simulink model "roach2_fengine_nlb"  (R2013b)
settings: Solver=VariableStepDiscrete  SolverMode=SingleTasking  StartTime=0.0  StopTime=10.0  RelTol=1e-3
undefined symbols (not defined in the file or in its folder): sfp
libraries: xbsIndex_r4 x3316, xps_library x74, casper_library_sources x16, casper_library_misc x7
(part 1 of 38)
settings Model: Creator=mdexter  LastModifiedBy=jackh
settings DataIOCC: SignalLoggingSaveFormat=ModelDataLogs
settings OptimizationCC: InlineParams=on  ExpressionDepthLimit=2147483647
settings DebuggingCC: FcnCallInpInsideContextMsg=UseLocalSettings  StateNameClashWarn=warning
settings GRTTargetCC: CombineOutputUpdateFcns=off  GRTInterface=on

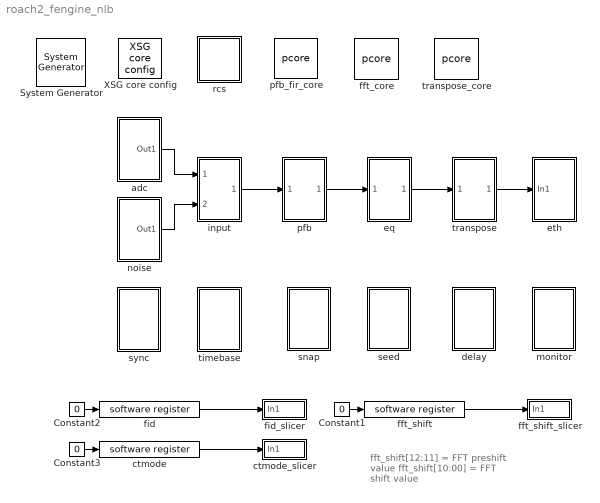
== system roach2_fengine_nlb ==
  note: fft_shift[12:11] = FFT preshift value
      | fft_shift[10:00] = FFT shift value
  " System Generator" : xbsIndex_r4/ System Generator  Tag=genX  xilinxfamily=virtex6  part=xc6vsx475t  speed=-1  package=ff1759  synthesis_tool=XST  clock_wrapper=Clock Enables  directory=./roach2_fengine/sysgen  proj_type=Project Navigator  Synth_file=XST Defaults  Impl_file=ISE Defaults  testbench=off  simulink_period=1  sysclk_period=5  dcm_input_clock_period=100  incr_netlist=off  trim_vbits=Everywhere in SubSystem  dbl_ovrd=According to Block Masks  core_generation=According to Block Masks  run_coregen=off  deprecated_control=off  eval_field=0  block_type=sysgen
      settings: block_version=10.1.3
  Constant1 : Constant  Value=0
  Constant2 : Constant  Value=0
  Constant3 : Constant  Value=0
  XSG core config : xps_library/XSG core config  Tag=xps:xsg  hw_sys=ROACH2:sx475t  clk_src=adc0_clk  ROACH_clk_src=adc0_clk  ROACH2_clk_src=adc0_clk  clk_rate=200  sample_period=1  synthesis_tool=XST
  adc : Subsystem
  ctmode : xps_library/software register  Tag=xps:sw_reg  io_dir=From Processor  arith_type=Unsigned  bitwidth=32  bin_pt=0  sample_period=1  gw_name=roach2_fengine_orig_ctmode_user_data_out
  ctmode_slicer : Subsystem
  delay : Subsystem
  eq : Subsystem
  eth : Subsystem
  fft_core : xps_library/pcore  Tag=xps:pcore  pcore_path=fft_1024ch_core/fft_1024ch_core.ngc
  fft_shift : xps_library/software register  Tag=xps:sw_reg  io_dir=From Processor  arith_type=Unsigned  bitwidth=32  bin_pt=0  sample_period=1  gw_name=roach2_fengine_orig_fft_shift_user_data_out
  fft_shift_slicer : Subsystem
  fid : xps_library/software register  Tag=xps:sw_reg  io_dir=From Processor  arith_type=Unsigned  bitwidth=32  bin_pt=0  sample_period=1  gw_name=roach2_fengine_orig_fid_user_data_out
  fid_slicer : Subsystem
  input : Subsystem
  monitor : Subsystem
  noise : Subsystem
  pfb : Subsystem
  pfb_fir_core : xps_library/pcore  Tag=xps:pcore  pcore_path=pfb_fir_1024ch_core/pfb_fir_1024ch_core.ngc
  rcs : Subsystem  AncestorBlock=casper_library_misc/rcs  mask(rcs){app_src=git, lib_src=git, user_val=0}
      mask prompts: app_src "Application revision info to capture"; lib_src "CASPER libraries revision info to capture"; user_val "User specified value"
      mask help:
      | Embeds revision control information for the user design and libraries.
      | On failure to locate specified revision information, falls back to
      | timestamps (current time for libraries).
      | A user specified value is also stored.
      mask init:
      | rcs_init(gcb, ...
      |     'app_src', app_src, ...
      |     'lib_src', lib_src);
      mask TypeOptions app_src: timestamp | git | svn
      mask TypeOptions lib_src: timestamp | git | svn
  seed : Subsystem
  snap : Subsystem
  sync : Subsystem
  timebase : Subsystem
  transpose : Subsystem
  transpose_core : xps_library/pcore  Tag=xps:pcore  pcore_path=transpose_core/transpose_core.ngc
  wires:
  input/1(Out1) -> pfb/1(In1)
  pfb/1(Out1) -> eq/1(In1)
  eq/1(Out2) -> transpose/1(In1)
  adc/1(Out1) -> input/1(In1)
  noise/1(Out1) -> input/2(In2)
  transpose/1(Out1) -> eth/1(In1)
  fft_shift/1 -> fft_shift_slicer/1(In1)
  Constant1/1 -> fft_shift/1
  fid/1 -> fid_slicer/1(In1)
  Constant2/1 -> fid/1
  ctmode/1 -> ctmode_slicer/1(In1)
  Constant3/1 -> ctmode/1

== system roach2_fengine_nlb/adc ==
  Bus Creator : BusCreator  Inputs=32
  Constant{3..34} (32 alike) : Constant  Value=0
  adc16x250-8 : Subsystem  Tag=xps:adc16  AncestorBlock=xps_library/ADCs/adc16x250-8  mask(ADC16){board_count=2, roach2_rev=2, zdok_rev=2}
      mask prompts: board_count "Number of ADC16 Boards"; roach2_rev "ROACH2 Revision"; zdok_rev "ZDOK Pinout Revision"
      mask help: 16-input ADC. When using one ADC16 board, it must be in ZDOK0.
      mask init:
      | % Only board_count is needed by init function
      | adc16_init(gcb, ...
      |     'board_count', board_count);
      settings: AttributesFormatString=r2 rev%<roach2_rev>\nzdok rev%<zdok_rev>
      mask Help:
      | This is the CASPER "yellow block" for the CASPER ADC16 board.  Each ADC
      | board has four ADC chips.  Each ADC chip accepts four inputs.  The four
      | 8-bit outputs from each ADC chip are concatenated into a 32-bit signal.
      mask TypeOptions board_count: 1 | 2
      mask TypeOptions roach2_rev: 1 | 2
      mask TypeOptions zdok_rev: 1 | 2
  Out1 : Outport
  wires:
  Constant3/1 -> adc16x250-8/1(a1_sim)
  Constant4/1 -> adc16x250-8/2(a2_sim)
  Constant5/1 -> adc16x250-8/3(a3_sim)
  Constant6/1 -> adc16x250-8/4(a4_sim)
  Constant7/1 -> adc16x250-8/5(b1_sim)
  Constant8/1 -> adc16x250-8/6(b2_sim)
  Constant9/1 -> adc16x250-8/7(b3_sim)
  Constant33/1 -> adc16x250-8/8(b4_sim)
  Constant34/1 -> adc16x250-8/9(c1_sim)
  Constant10/1 -> adc16x250-8/10(c2_sim)
  Constant11/1 -> adc16x250-8/11(c3_sim)
  Constant12/1 -> adc16x250-8/12(c4_sim)
  Constant13/1 -> adc16x250-8/13(d1_sim)
  Constant14/1 -> adc16x250-8/14(d2_sim)
  Constant15/1 -> adc16x250-8/15(d3_sim)
  Constant17/1 -> adc16x250-8/16(d4_sim)
  Constant16/1 -> adc16x250-8/17(e1_sim)
  Constant25/1 -> adc16x250-8/18(e2_sim)
  Constant26/1 -> adc16x250-8/19(e3_sim)
  Constant27/1 -> adc16x250-8/20(e4_sim)
  Constant28/1 -> adc16x250-8/21(f1_sim)
  Constant29/1 -> adc16x250-8/22(f2_sim)
  Constant30/1 -> adc16x250-8/23(f3_sim)
  Constant31/1 -> adc16x250-8/24(f4_sim)
  Constant32/1 -> adc16x250-8/25(g1_sim)
  Constant18/1 -> adc16x250-8/26(g2_sim)
  Constant19/1 -> adc16x250-8/27(g3_sim)
  Constant20/1 -> adc16x250-8/28(g4_sim)
  Constant21/1 -> adc16x250-8/29(h1_sim)
  Constant22/1 -> adc16x250-8/30(h2_sim)
  Constant23/1 -> adc16x250-8/31(h3_sim)
  Constant24/1 -> adc16x250-8/32(h4_sim)
  Bus Creator/1 -> Out1/1
  adc16x250-8/1(a1) -> Bus Creator/1
  adc16x250-8/2(a2) -> Bus Creator/2
  adc16x250-8/3(a3) -> Bus Creator/3
  adc16x250-8/4(a4) -> Bus Creator/4
  adc16x250-8/5(b1) -> Bus Creator/5
  adc16x250-8/6(b2) -> Bus Creator/6
  adc16x250-8/7(b3) -> Bus Creator/7
  adc16x250-8/8(b4) -> Bus Creator/8
  adc16x250-8/9(c1) -> Bus Creator/9
  adc16x250-8/10(c2) -> Bus Creator/10
  adc16x250-8/11(c3) -> Bus Creator/11
  adc16x250-8/12(c4) -> Bus Creator/12
  adc16x250-8/13(d1) -> Bus Creator/13
  adc16x250-8/14(d2) -> Bus Creator/14
  adc16x250-8/15(d3) -> Bus Creator/15
  adc16x250-8/16(d4) -> Bus Creator/16
  adc16x250-8/17(e1) -> Bus Creator/17
  adc16x250-8/18(e2) -> Bus Creator/18
  adc16x250-8/19(e3) -> Bus Creator/19
  adc16x250-8/20(e4) -> Bus Creator/20
  adc16x250-8/21(f1) -> Bus Creator/21
  adc16x250-8/22(f2) -> Bus Creator/22
  adc16x250-8/23(f3) -> Bus Creator/23
  adc16x250-8/24(f4) -> Bus Creator/24
  adc16x250-8/25(g1) -> Bus Creator/25
  adc16x250-8/26(g2) -> Bus Creator/26
  adc16x250-8/27(g3) -> Bus Creator/27
  adc16x250-8/28(g4) -> Bus Creator/28
  adc16x250-8/29(h1) -> Bus Creator/29
  adc16x250-8/30(h2) -> Bus Creator/30
  adc16x250-8/31(h3) -> Bus Creator/31
  adc16x250-8/32(h4) -> Bus Creator/32

== system roach2_fengine_nlb/ctmode_slicer ==
  In1 : Inport
  Delay8 : xbsIndex_r4/Delay  rst=off  infoeditControl=Selection of Reset will increase slice count due to use of real FFs and instead of SRLs  en=off  latency=2  dbl_ovrd=off  reg_retiming=on  block_type=delay
      settings: xl_area=[0, 0, 0, 0, 0, 0, 0]
  b1_b0 : xbsIndex_r4/Slice  nbits=2  boolean_output=off  mode=Lower Bit Location + Width  bit1=0  base1=MSB of Input  bit0=0  base0=LSB of Input  dbl_ovrd=off  block_type=slice
      settings: block_version=10.1.3
  tag scope: ctmode=global
  wires:
  Delay8/1 -> b1_b0/1
  b1_b0/1 -> [ctmode]
  In1/1 -> Delay8/1

== system roach2_fengine_nlb/delay ==
  0 : xps_library/software register  Tag=xps:sw_reg  io_dir=From Processor  arith_type=Unsigned  bitwidth=32  bin_pt=0  sample_period=1  gw_name=roach2_fengine_delay_0_user_data_out
  1 : xps_library/software register  Tag=xps:sw_reg  io_dir=From Processor  arith_type=Unsigned  bitwidth=32  bin_pt=0  sample_period=1  gw_name=roach2_fengine_delay_1_user_data_out
  2 : xps_library/software register  Tag=xps:sw_reg  io_dir=From Processor  arith_type=Unsigned  bitwidth=32  bin_pt=0  sample_period=1  gw_name=roach2_fengine_delay_2_user_data_out
  3 : xps_library/software register  Tag=xps:sw_reg  io_dir=From Processor  arith_type=Unsigned  bitwidth=32  bin_pt=0  sample_period=1  gw_name=roach2_fengine_delay_3_user_data_out
  4 : xps_library/software register  Tag=xps:sw_reg  io_dir=From Processor  arith_type=Unsigned  bitwidth=32  bin_pt=0  sample_period=1  gw_name=roach2_fengine_delay_4_user_data_out
  5 : xps_library/software register  Tag=xps:sw_reg  io_dir=From Processor  arith_type=Unsigned  bitwidth=32  bin_pt=0  sample_period=1  gw_name=roach2_fengine_delay_5_user_data_out
  6 : xps_library/software register  Tag=xps:sw_reg  io_dir=From Processor  arith_type=Unsigned  bitwidth=32  bin_pt=0  sample_period=1  gw_name=roach2_fengine_delay_6_user_data_out
  7 : xps_library/software register  Tag=xps:sw_reg  io_dir=From Processor  arith_type=Unsigned  bitwidth=32  bin_pt=0  sample_period=1  gw_name=roach2_fengine_delay_7_user_data_out
  BitBasher : xbsIndex_r4/BitBasher  bitexpr=|  display_expr=off  sr_1=1  arith_type1=Unsigned  bin_pt1=0  sr_2=2  arith_type2=Unsigned  bin_pt2=0  sr_3=3  arith_type3=Unsigned  bin_pt3=0  sr_4=4  arith_type4=Unsigned  bin_pt4=0  dbl_ovrd=off  block_type=bitbasher
      | <!DOCTYPE HTML PUBLIC "-//W3C//DTD HTML 4.0//EN" "http://www.w3.org/TR/REC-html40/strict.dtd">
      | <html><head><meta name="qrichtext" content="1" /><style type="text/css">
      | p, li { white-space: pre-wrap; }
      | </style></head><body style=" font-family:'Sans'; font-size:10pt; font-weight:400; font-style:normal;">
      | <p style=" margin-top:12px; margin-bottom:12px; margin-left:0px; margin-right:0px; -qt-block-indent:0; text-indent:0px;"><span style=" font-family:'MS Shell Dlg'; font-size:8pt;">d={b,a}</span></p></body></html>
  BitBasher1 : xbsIndex_r4/BitBasher  bitexpr=|  display_expr=off  sr_1=1  arith_type1=Unsigned  bin_pt1=0  sr_2=2  arith_type2=Unsigned  bin_pt2=0  sr_3=3  arith_type3=Unsigned  bin_pt3=0  sr_4=4  arith_type4=Unsigned  bin_pt4=0  dbl_ovrd=off  block_type=bitbasher
      | <!DOCTYPE HTML PUBLIC "-//W3C//DTD HTML 4.0//EN" "http://www.w3.org/TR/REC-html40/strict.dtd">
      | <html><head><meta name="qrichtext" content="1" /><style type="text/css">
      | p, li { white-space: pre-wrap; }
      | </style></head><body style=" font-family:'Sans'; font-size:10pt; font-weight:400; font-style:normal;">
      | <p style=" margin-top:12px; margin-bottom:12px; margin-left:0px; margin-right:0px; -qt-block-indent:0; text-indent:0px;"><span style=" font-family:'MS Shell Dlg'; font-size:8pt;">d={b,a}</span></p></body></html>
  BitBasher2 : xbsIndex_r4/BitBasher  bitexpr=|  display_expr=off  sr_1=1  arith_type1=Unsigned  bin_pt1=0  sr_2=2  arith_type2=Unsigned  bin_pt2=0  sr_3=3  arith_type3=Unsigned  bin_pt3=0  sr_4=4  arith_type4=Unsigned  bin_pt4=0  dbl_ovrd=off  block_type=bitbasher
      | <!DOCTYPE HTML PUBLIC "-//W3C//DTD HTML 4.0//EN" "http://www.w3.org/TR/REC-html40/strict.dtd">
      | <html><head><meta name="qrichtext" content="1" /><style type="text/css">
      | p, li { white-space: pre-wrap; }
      | </style></head><body style=" font-family:'Sans'; font-size:10pt; font-weight:400; font-style:normal;">
      | <p style=" margin-top:12px; margin-bottom:12px; margin-left:0px; margin-right:0px; -qt-block-indent:0; text-indent:0px;"><span style=" font-family:'MS Shell Dlg'; font-size:8pt;">d={b,a}</span></p></body></html>
  BitBasher3 : xbsIndex_r4/BitBasher  bitexpr=|  display_expr=off  sr_1=1  arith_type1=Unsigned  bin_pt1=0  sr_2=2  arith_type2=Unsigned  bin_pt2=0  sr_3=3  arith_type3=Unsigned  bin_pt3=0  sr_4=4  arith_type4=Unsigned  bin_pt4=0  dbl_ovrd=off  block_type=bitbasher
      | <!DOCTYPE HTML PUBLIC "-//W3C//DTD HTML 4.0//EN" "http://www.w3.org/TR/REC-html40/strict.dtd">
      | <html><head><meta name="qrichtext" content="1" /><style type="text/css">
      | p, li { white-space: pre-wrap; }
      | </style></head><body style=" font-family:'Sans'; font-size:10pt; font-weight:400; font-style:normal;">
      | <p style=" margin-top:12px; margin-bottom:12px; margin-left:0px; margin-right:0px; -qt-block-indent:0; text-indent:0px;"><span style=" font-family:'MS Shell Dlg'; font-size:8pt;">d={b,a}</span></p></body></html>
  Constant{,1..7} (8 alike) : Constant  Value=0
  tag scope: delay0=global, delay1=global, delay2=global, delay3=global
  wires:
  0/1 -> BitBasher/1
  Constant/1 -> 0/1
  1/1 -> BitBasher/2
  Constant1/1 -> 1/1
  2/1 -> BitBasher1/1
  Constant2/1 -> 2/1
  3/1 -> BitBasher1/2
  Constant3/1 -> 3/1
  4/1 -> BitBasher2/1
  Constant4/1 -> 4/1
  5/1 -> BitBasher2/2
  Constant5/1 -> 5/1
  6/1 -> BitBasher3/1
  Constant6/1 -> 6/1
  7/1 -> BitBasher3/2
  Constant7/1 -> 7/1
  BitBasher/1 -> [delay0]
  BitBasher1/1 -> [delay1]
  BitBasher2/1 -> [delay2]
  BitBasher3/1 -> [delay3]

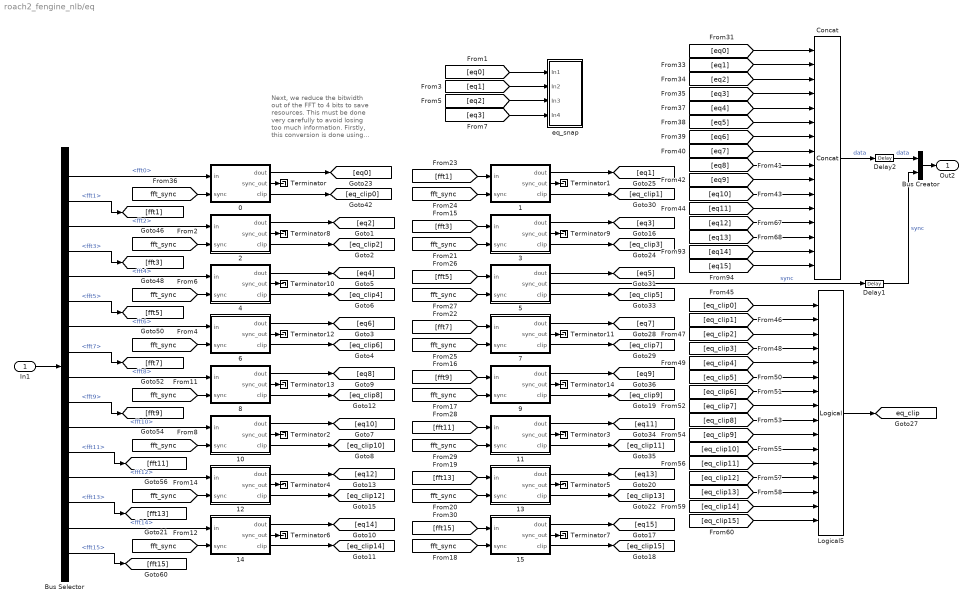
== system roach2_fengine_nlb/eq ==
  note: Next, we reduce the bitwidth out of the FFT to 4 bits to save resources.
      | This must be done very carefully to avoid losing too much information.
      | Firstly, this conversion is done using "Round to Even" and saturation
      | logic to avoid introducing DC offsets, wrapping, and other ugly quantizaton
      | effects.  Secondly, the "equalizer" allows each frequency channel of the
      | FFT to be scaled by a different number.  This allows passbands which are
      | not flat to be flattened digitally to allow for optimal quantization to 4 bits.
      | These coefficients can also be updated dynamically for gain control.
      | Coefficients can be dynamically written into the "equalizer" by
      | specifying the channel ("coeff_addr") and the value of the
      | coefficient ("coeff"), and then using "coeff_en" to write the
      | new coefficient into the equalization table.
  In1 : Inport
  0 : Subsystem  mask{nchan=11}
      mask prompts: nchan "Number of fft channels (same as fft prompt) (2^?)"
  1 : Subsystem  mask{nchan=11}
      mask prompts: nchan "Number of fft channels (same as fft prompt) (2^?)"
  10 : Subsystem  mask{nchan=11}
      mask prompts: nchan "Number of fft channels (same as fft prompt) (2^?)"
  11 : Subsystem  mask{nchan=11}
      mask prompts: nchan "Number of fft channels (same as fft prompt) (2^?)"
  12 : Subsystem  mask{nchan=11}
      mask prompts: nchan "Number of fft channels (same as fft prompt) (2^?)"
  13 : Subsystem  mask{nchan=11}
      mask prompts: nchan "Number of fft channels (same as fft prompt) (2^?)"
  14 : Subsystem  mask{nchan=11}
      mask prompts: nchan "Number of fft channels (same as fft prompt) (2^?)"
  15 : Subsystem  mask{nchan=11}
      mask prompts: nchan "Number of fft channels (same as fft prompt) (2^?)"
  2 : Subsystem  mask{nchan=11}
      mask prompts: nchan "Number of fft channels (same as fft prompt) (2^?)"
  3 : Subsystem  mask{nchan=11}
      mask prompts: nchan "Number of fft channels (same as fft prompt) (2^?)"
  4 : Subsystem  mask{nchan=11}
      mask prompts: nchan "Number of fft channels (same as fft prompt) (2^?)"
  5 : Subsystem  mask{nchan=11}
      mask prompts: nchan "Number of fft channels (same as fft prompt) (2^?)"
  6 : Subsystem  mask{nchan=11}
      mask prompts: nchan "Number of fft channels (same as fft prompt) (2^?)"
  7 : Subsystem  mask{nchan=11}
      mask prompts: nchan "Number of fft channels (same as fft prompt) (2^?)"
  8 : Subsystem  mask{nchan=11}
      mask prompts: nchan "Number of fft channels (same as fft prompt) (2^?)"
  9 : Subsystem  mask{nchan=11}
      mask prompts: nchan "Number of fft channels (same as fft prompt) (2^?)"
  Bus Creator : BusCreator  Inputs=2
  Bus Selector : BusSelector  OutputSignals=fft0,fft1,fft2,fft3,fft4,fft5,fft6,fft7,fft8,fft9,fft10,fft11,fft12,fft13,fft14,fft15
  Concat : xbsIndex_r4/Concat  num_inputs=16  dbl_ovrd=off  block_type=concat
  Delay1 : xbsIndex_r4/Delay  rst=off  infoeditControl=Selection of Reset will increase slice count due to use of real FFs and instead of SRLs  en=off  latency=1  dbl_ovrd=off  reg_retiming=off  block_type=delay
  Delay2 : xbsIndex_r4/Delay  rst=off  infoeditControl=Selection of Reset will increase slice count due to use of real FFs and instead of SRLs  en=off  latency=1  dbl_ovrd=off  reg_retiming=off  block_type=delay
  Logical5 : xbsIndex_r4/Logical  logical_function=OR  inputs=16  en=off  latency=1  precision=Full  arith_type=Unsigned  n_bits=8  bin_pt=2  align_bp=on  dbl_ovrd=off  block_type=logical
      settings: xl_area=[0, 0, 0, 0, 0, 0, 0]
  Terminator{,1..14} (15 alike) : Terminator
  eq_snap : Subsystem
  Out2 : Outport
  tag scope: eq_clip=global
  wires:
  0/1(dout) -> [eq0]
  0/3(clip) -> [eq_clip0]
  Logical5/1 -> [eq_clip]
  [fft_sync] -> 0/2(sync)
  Delay2/1 -> Bus Creator/1  "data"
  Bus Creator/1 -> Out2/1
  2/1(dout) -> [eq2]
  2/3(clip) -> [eq_clip2]
  [fft_sync] -> 2/2(sync)
  4/1(dout) -> [eq4]
  Bus Selector/5 -> 4/1(in)  "<fft4>"
  4/3(clip) -> [eq_clip4]
  [fft_sync] -> 4/2(sync)
  6/1(dout) -> [eq6]
  Bus Selector/7 -> 6/1(in)  "<fft6>"
  6/3(clip) -> [eq_clip6]
  [fft_sync] -> 6/2(sync)
  8/1(dout) -> [eq8]
  Bus Selector/9 -> 8/1(in)  "<fft8>"
  8/3(clip) -> [eq_clip8]
  [fft_sync] -> 8/2(sync)
  10/1(dout) -> [eq10]
  Bus Selector/11 -> 10/1(in)  "<fft10>"
  10/3(clip) -> [eq_clip10]
  [fft_sync] -> 10/2(sync)
  12/1(dout) -> [eq12]
  Bus Selector/13 -> 12/1(in)  "<fft12>"
  12/3(clip) -> [eq_clip12]
  [fft_sync] -> 12/2(sync)
  14/1(dout) -> [eq14]
  Bus Selector/15 -> 14/1(in)  "<fft14>"
  14/3(clip) -> [eq_clip14]
  [fft_sync] -> 14/2(sync)
  1/1(dout) -> [eq1]
  1/3(clip) -> [eq_clip1]
  [fft_sync] -> 1/2(sync)
  3/1(dout) -> [eq3]
  [fft3] -> 3/1(in)
  3/3(clip) -> [eq_clip3]
  [fft_sync] -> 3/2(sync)
  5/1(dout) -> [eq5]
  [fft5] -> 5/1(in)
  5/3(clip) -> [eq_clip5]
  [fft_sync] -> 5/2(sync)
  7/1(dout) -> [eq7]
  [fft7] -> 7/1(in)
  7/3(clip) -> [eq_clip7]
  [fft_sync] -> 7/2(sync)
  9/1(dout) -> [eq9]
  [fft9] -> 9/1(in)
  9/3(clip) -> [eq_clip9]
  [fft_sync] -> 9/2(sync)
  11/1(dout) -> [eq11]
  [fft11] -> 11/1(in)
  11/3(clip) -> [eq_clip11]
  [fft_sync] -> 11/2(sync)
  13/1(dout) -> [eq13]
  [fft13] -> 13/1(in)
  13/3(clip) -> [eq_clip13]
  [fft_sync] -> 13/2(sync)
  15/1(dout) -> [eq15]
  [fft15] -> 15/1(in)
  15/3(clip) -> [eq_clip15]
  [fft_sync] -> 15/2(sync)
  [eq0] -> Concat/1
  [eq1] -> Concat/2
  [eq2] -> Concat/3
  [eq3] -> Concat/4
  [eq4] -> Concat/5
  [eq5] -> Concat/6
  [eq6] -> Concat/7
  [eq7] -> Concat/8
  [eq8] -> Concat/9
  [eq9] -> Concat/10
  [eq10] -> Concat/11
  [eq11] -> Concat/12
  [eq12] -> Concat/13
  [eq13] -> Concat/14
  [eq14] -> Concat/15
  [eq15] -> Concat/16
  [eq_clip0] -> Logical5/1
  [eq_clip1] -> Logical5/2
  [eq_clip2] -> Logical5/3
  [eq_clip3] -> Logical5/4
  [eq_clip4] -> Logical5/5
  [eq_clip5] -> Logical5/6
  [eq_clip6] -> Logical5/7
  [eq_clip7] -> Logical5/8
  [eq_clip8] -> Logical5/9
  [eq_clip9] -> Logical5/10
  [eq_clip10] -> Logical5/11
  [eq_clip11] -> Logical5/12
  [eq_clip12] -> Logical5/13
  [eq_clip13] -> Logical5/14
  [eq_clip14] -> Logical5/15
  [eq_clip15] -> Logical5/16
  In1/1 -> Bus Selector/1
  Bus Selector/1 -> 0/1(in)  "<fft0>"
  Bus Selector/3 -> 2/1(in)  "<fft2>"
  [fft1] -> 1/1(in)
  Bus Selector/16 -> [fft15]  "<fft15>"
  Bus Selector/14 -> [fft13]  "<fft13>"
  Bus Selector/12 -> [fft11]  "<fft11>"
  Bus Selector/10 -> [fft9]  "<fft9>"
  Bus Selector/8 -> [fft7]  "<fft7>"
  Bus Selector/6 -> [fft5]  "<fft5>"
  Bus Selector/4 -> [fft3]  "<fft3>"
  Bus Selector/2 -> [fft1]  "<fft1>"
  0/2(sync_out) -> Terminator/1
  1/2(sync_out) -> Terminator1/1
  10/2(sync_out) -> Terminator2/1
  11/2(sync_out) -> Terminator3/1
  12/2(sync_out) -> Terminator4/1
  13/2(sync_out) -> Terminator5/1
  14/2(sync_out) -> Terminator6/1
  15/2(sync_out) -> Terminator7/1
  2/2(sync_out) -> Terminator8/1
  3/2(sync_out) -> Terminator9/1
  4/2(sync_out) -> Terminator10/1
  5/2(sync_out) -> Delay1/1  "sync"
  6/2(sync_out) -> Terminator12/1
  8/2(sync_out) -> Terminator13/1
  9/2(sync_out) -> Terminator14/1
  7/2(sync_out) -> Terminator11/1
  Concat/1 -> Delay2/1  "data"
  Delay1/1 -> Bus Creator/2  "sync"
  [eq0] -> eq_snap/1(In1)
  [eq1] -> eq_snap/2(In2)
  [eq2] -> eq_snap/3(In3)
  [eq3] -> eq_snap/4(In4)

== system roach2_fengine_nlb/eth ==
  note: IP and MAC address assignments for ports connected to switch
      | eth0: IP=10.10.10.(32+FID)  MAC=02:02:0A:0A:0A:(20+FID)
      | eth1: IP=10.10.10.(40+FID)  MAC=02:02:0A:0A:0A:(28+FID)
      | eth2: IP=10.10.10.(48+FID)  MAC=02:02:0A:0A:0A:(30+FID)
      | eth3: IP=10.10.10.(56+FID)  MAC=02:02:0A:0A:0A:(38+FID)
  note: IP and MAC address assignments for ports connected to GPU X engines
      | eth0: IP=192.168.2.(1+FID)  MAC=02:02:C0:A8:02:(1+FID)
      | eth1: IP=192.168.3.(1+FID)  MAC=02:02:C0:A8:03:(1+FID)
      | eth2: IP=192.168.4.(1+FID)  MAC=02:02:C0:A8:04:(1+FID)
      | eth3: IP=192.168.5.(1+FID)  MAC=02:02:C0:A8:05:(1+FID)
  note: ctrl[8] = cnt_rst
      | ctrl[5] = gbe_gpu_rst
      | ctrl[4] = gbe_sw_rdst
      | ctrl[1] = gbe_gpu_en
      | ctrl[0] = gbe_sw_en
  In1 : Inport
  0 : Subsystem
  1 : Subsystem
  2 : Subsystem
  3 : Subsystem
  BitBasher : xbsIndex_r4/BitBasher  bitexpr=|  display_expr=off  sr_1=1  arith_type1=Unsigned  bin_pt1=0  sr_2=2  arith_type2=Unsigned  bin_pt2=0  sr_3=3  arith_type3=Unsigned  bin_pt3=0  sr_4=4  arith_type4=Unsigned  bin_pt4=0  dbl_ovrd=off  block_type=bitbasher
      | <!DOCTYPE HTML PUBLIC "-//W3C//DTD HTML 4.0//EN" "http://www.w3.org/TR/REC-html40/strict.dtd">
      | <html><head><meta name="qrichtext" content="1" /><style type="text/css">
      | p, li { white-space: pre-wrap; }
      | </style></head><body style=" font-family:'Sans'; font-size:10pt; font-weight:400; font-style:normal;">
      | <p style=" margin-top:12px; margin-bottom:12px; margin-left:0px; margin-right:0px; -qt-block-indent:0; text-indent:0px;"><span style=" font-family:'MS Shell Dlg'; font-size:8pt;">gpurst={ctrl[5]}<br />swrst={ctrl[4]}<br />gpuen={ctrl[1]}<br />swen={ctrl[0]}</span></p></body></html>
  BitBasher1 : xbsIndex_r4/BitBasher  bitexpr=|  display_expr=off  sr_1=1  arith_type1=Unsigned  bin_pt1=0  sr_2=2  arith_type2=Unsigned  bin_pt2=0  sr_3=3  arith_type3=Unsigned  bin_pt3=0  sr_4=4  arith_type4=Unsigned  bin_pt4=0  dbl_ovrd=off  block_type=bitbasher
      | <!DOCTYPE HTML PUBLIC "-//W3C//DTD HTML 4.0//EN" "http://www.w3.org/TR/REC-html40/strict.dtd">
      | <html><head><meta name="qrichtext" content="1" /><style type="text/css">
      | p, li { white-space: pre-wrap; }
      | </style></head><body style=" font-family:'Sans'; font-size:10pt; font-weight:400; font-style:normal;">
      | <p style=" margin-top:12px; margin-bottom:12px; margin-left:0px; margin-right:0px; -qt-block-indent:0; text-indent:0px;"><span style=" font-family:'MS Shell Dlg'; font-size:8pt;">cntrst={ctrl[8]}<br /></span></p></body></html>
  Bus Selector2 : BusSelector  OutputSignals=chan_0_255,chan_256_511,chan_512_767,chan_768_1023
  Constant1 : Constant  Value=0
  Constant3 : xbsIndex_r4/Constant  const=0  gui_display_data_type=Fixed-point  arith_type=Unsigned  n_bits=2  bin_pt=0  preci_type=Single  exp_width=8  frac_width=24  explicit_period=on  period=1  equ=P=C  opselect=C  inp2=PCIN>>17  opr=+  inp1=P  carry=CIN  dbl_ovrd=off  block_type=constant
  Constant5 : xbsIndex_r4/Constant  const=1  gui_display_data_type=Fixed-point  arith_type=Unsigned  n_bits=2  bin_pt=0  preci_type=Single  exp_width=8  frac_width=24  explicit_period=on  period=1  equ=P=C  opselect=C  inp2=PCIN>>17  opr=+  inp1=P  carry=CIN  dbl_ovrd=off  block_type=constant
  Constant7 : xbsIndex_r4/Constant  const=2  gui_display_data_type=Fixed-point  arith_type=Unsigned  n_bits=2  bin_pt=0  preci_type=Single  exp_width=8  frac_width=24  explicit_period=on  period=1  equ=P=C  opselect=C  inp2=PCIN>>17  opr=+  inp1=P  carry=CIN  dbl_ovrd=off  block_type=constant
  Constant8 : xbsIndex_r4/Constant  const=3  gui_display_data_type=Fixed-point  arith_type=Unsigned  n_bits=2  bin_pt=0  preci_type=Single  exp_width=8  frac_width=24  explicit_period=on  period=1  equ=P=C  opselect=C  inp2=PCIN>>17  opr=+  inp1=P  carry=CIN  dbl_ovrd=off  block_type=constant
  Convert{1..4} (4 alike) : xbsIndex_r4/Convert  gui_display_data_type=Boolean  arith_type=Boolean  n_bits=32  bin_pt=0  float_type=Single  exp_bits=8  fraction_bits=24  quantization=Truncate  overflow=Wrap  en=off  latency=0  dbl_ovrd=off  pipeline=off  block_type=convert
      settings: block_version=11.4
  Delay2 : xbsIndex_r4/Delay  rst=off  infoeditControl=Selection of Reset will increase slice count due to use of real FFs and instead of SRLs  en=off  latency=2  dbl_ovrd=off  reg_retiming=on  block_type=delay
  ctrl : xps_library/software register  Tag=xps:sw_reg  io_dir=From Processor  arith_type=Unsigned  bitwidth=32  bin_pt=0  sample_period=1  gw_name=roach2_fengine_orig_eth_ctrl_user_data_out
  tag scope: cnt_rst=global, gbe_gpu_en=global, gbe_gpu_rst=global, gbe_sw_en=global, gbe_sw_rst=global
  wires:
  Constant5/1 -> 0/2(sw_base)
  In1/1 -> Bus Selector2/1
  [chan_256_511] -> 0/1(data)
  Bus Selector2/1 -> [chan_0_255]  "<chan_0_255>"
  Bus Selector2/2 -> [chan_256_511]  "<chan_256_511>"
  Bus Selector2/3 -> [chan_512_767]  "<chan_512_767>"
  Bus Selector2/4 -> [chan_768_1023]  "<chan_768_1023>"
  Constant3/1 -> 1/2(sw_base)
  [chan_0_255] -> 1/1(data)
  Constant8/1 -> 2/2(sw_base)
  [chan_768_1023] -> 2/1(data)
  Constant7/1 -> 3/2(sw_base)
  [chan_512_767] -> 3/1(data)
  Constant1/1 -> ctrl/1
  BitBasher/1 -> Convert2/1
  BitBasher/2 -> Convert3/1
  BitBasher/3 -> Convert4/1
  BitBasher/4 -> [gbe_sw_en]
  BitBasher1/1 -> Convert1/1
  Convert2/1 -> [gbe_gpu_rst]
  Convert1/1 -> [cnt_rst]
  Convert3/1 -> [gbe_sw_rst]
  Convert4/1 -> [gbe_gpu_en]
  ctrl/1 -> Delay2/1
  Delay2/1 -> BitBasher/1, BitBasher1/1

== system roach2_fengine_nlb/fft_shift_slicer ==
  In1 : Inport
  Convert : xbsIndex_r4/Convert  gui_display_data_type=Fixed-point  arith_type=Unsigned  n_bits=16  bin_pt=0  float_type=Single  exp_bits=8  fraction_bits=24  quantization=Truncate  overflow=Wrap  en=off  latency=0  dbl_ovrd=off  pipeline=off  block_type=convert
  Delay8 : xbsIndex_r4/Delay  rst=off  infoeditControl=Selection of Reset will increase slice count due to use of real FFs and instead of SRLs  en=off  latency=2  dbl_ovrd=off  reg_retiming=on  block_type=delay
      settings: xl_area=[0, 0, 0, 0, 0, 0, 0]
  b10_b0 : xbsIndex_r4/Slice  nbits=11  boolean_output=off  mode=Lower Bit Location + Width  bit1=0  base1=MSB of Input  bit0=0  base0=LSB of Input  dbl_ovrd=off  block_type=slice
      settings: block_version=10.1.3
  b12_b11 : xbsIndex_r4/Slice  nbits=2  boolean_output=off  mode=Lower Bit Location + Width  bit1=0  base1=MSB of Input  bit0=11  base0=LSB of Input  dbl_ovrd=off  block_type=slice
      settings: block_version=10.1.3
  tag scope: fft_preshift=global, fft_shift=global
  wires:
  Delay8/1 -> b10_b0/1, b12_b11/1
  b10_b0/1 -> Convert/1
  b12_b11/1 -> [fft_preshift]
  In1/1 -> Delay8/1
  Convert/1 -> [fft_shift]

== system roach2_fengine_nlb/fid_slicer ==
  In1 : Inport
  Delay8 : xbsIndex_r4/Delay  rst=off  infoeditControl=Selection of Reset will increase slice count due to use of real FFs and instead of SRLs  en=off  latency=2  dbl_ovrd=off  reg_retiming=on  block_type=delay
      settings: xl_area=[0, 0, 0, 0, 0, 0, 0]
  b2_b0 : xbsIndex_r4/Slice  nbits=3  boolean_output=off  mode=Lower Bit Location + Width  bit1=0  base1=MSB of Input  bit0=0  base0=LSB of Input  dbl_ovrd=off  block_type=slice
      settings: block_version=10.1.3
  tag scope: FID=global
  wires:
  Delay8/1 -> b2_b0/1
  b2_b0/1 -> [FID]
  In1/1 -> Delay8/1

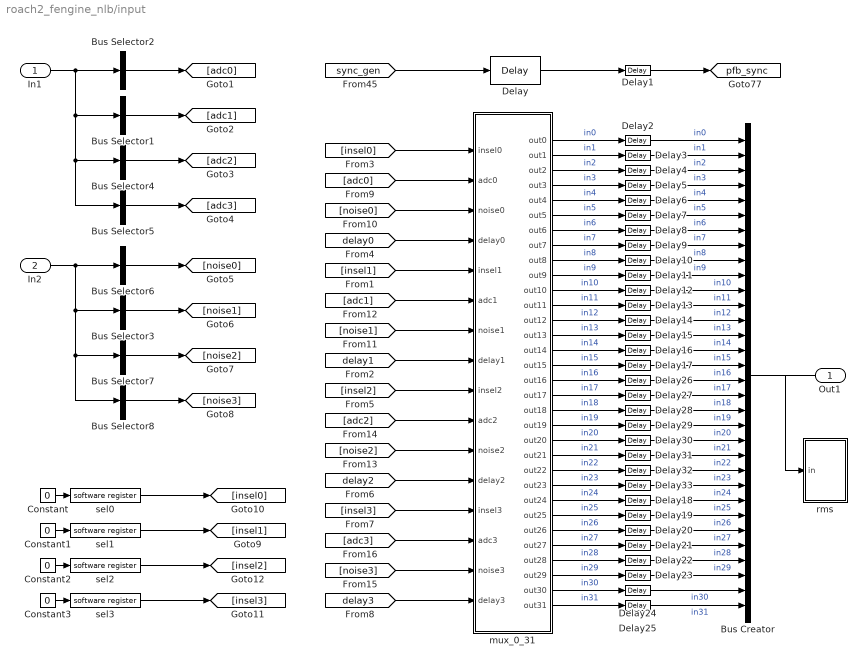
== system roach2_fengine_nlb/input ==
  In1 : Inport
  In2 : Inport  Port=2
  Bus Creator : BusCreator  Inputs=32
  Bus Selector1 : BusSelector  OutputSignals=c1,c2,c3,c4,d1,d2,d3,d4  OutputAsBus=on
  Bus Selector2 : BusSelector  OutputSignals=a1,a2,a3,a4,b1,b2,b3,b4  OutputAsBus=on
  Bus Selector3 : BusSelector  OutputSignals=n8,n9,n10,n11,n12,n13,n14,n15  OutputAsBus=on
  Bus Selector4 : BusSelector  OutputSignals=e1,e2,e3,e4,f1,f2,f3,f4  OutputAsBus=on
  Bus Selector5 : BusSelector  OutputSignals=g1,g2,g3,g4,h1,h2,h3,h4  OutputAsBus=on
  Bus Selector6 : BusSelector  OutputSignals=n0,n1,n2,n3,n4,n5,n6,n7  OutputAsBus=on
  Bus Selector7 : BusSelector  OutputSignals=n16,n17,n18,n19,n20,n21,n22,n23  OutputAsBus=on
  Bus Selector8 : BusSelector  OutputSignals=n24,n25,n26,n27,n28,n29,n30,n31  OutputAsBus=on
  Constant{,1..3} (4 alike) : Constant  Value=0
  Delay : xbsIndex_r4/Delay  rst=off  infoeditControl=Selection of Reset will increase slice count due to use of real FFs and instead of SRLs  en=off  latency=2  dbl_ovrd=off  reg_retiming=off  block_type=delay
  Delay{1..33} (33 alike) : xbsIndex_r4/Delay  rst=off  infoeditControl=Selection of Reset will increase slice count due to use of real FFs and instead of SRLs  en=off  latency=1  dbl_ovrd=off  reg_retiming=off  block_type=delay
  mux_0_31 : Subsystem
  rms : Subsystem
  sel0 : xps_library/software register  Tag=xps:sw_reg  io_dir=From Processor  arith_type=Unsigned  bitwidth=32  bin_pt=0  sample_period=1  gw_name=roach2_fengine_input_sel0_user_data_out
  sel1 : xps_library/software register  Tag=xps:sw_reg  io_dir=From Processor  arith_type=Unsigned  bitwidth=32  bin_pt=0  sample_period=1  gw_name=roach2_fengine_input_sel1_user_data_out
  sel2 : xps_library/software register  Tag=xps:sw_reg  io_dir=From Processor  arith_type=Unsigned  bitwidth=32  bin_pt=0  sample_period=1  gw_name=roach2_fengine_input_sel2_user_data_out
  sel3 : xps_library/software register  Tag=xps:sw_reg  io_dir=From Processor  arith_type=Unsigned  bitwidth=32  bin_pt=0  sample_period=1  gw_name=roach2_fengine_input_sel3_user_data_out
  Out1 : Outport
  tag scope: pfb_sync=global
  wires:
  [sync_gen] -> Delay/1
  Delay/1 -> Delay1/1
  [insel0] -> mux_0_31/1(insel0)
  [delay0] -> mux_0_31/4(delay0)
  [insel1] -> mux_0_31/5(insel1)
  [delay1] -> mux_0_31/8(delay1)
  [insel2] -> mux_0_31/9(insel2)
  [delay2] -> mux_0_31/12(delay2)
  [insel3] -> mux_0_31/13(insel3)
  [delay3] -> mux_0_31/16(delay3)
  In1/1 -> Bus Selector2/1, Bus Selector1/1, Bus Selector5/1, Bus Selector4/1
  Bus Selector2/1 -> [adc0]
  [adc0] -> mux_0_31/2(adc0)
  [noise0] -> mux_0_31/3(noise0)
  [adc1] -> mux_0_31/6(adc1)
  [noise1] -> mux_0_31/7(noise1)
  [adc2] -> mux_0_31/10(adc2)
  [noise2] -> mux_0_31/11(noise2)
  [adc3] -> mux_0_31/14(adc3)
  [noise3] -> mux_0_31/15(noise3)
  Bus Selector1/1 -> [adc1]
  Bus Selector4/1 -> [adc2]
  Bus Selector5/1 -> [adc3]
  In2/1 -> Bus Selector6/1, Bus Selector3/1, Bus Selector8/1, Bus Selector7/1
  Bus Selector6/1 -> [noise0]
  Bus Selector3/1 -> [noise1]
  Bus Selector7/1 -> [noise2]
  Bus Selector8/1 -> [noise3]
  Bus Creator/1 -> Out1/1, rms/1(in)
  Delay2/1 -> Bus Creator/1  "in0"
  Delay3/1 -> Bus Creator/2  "in1"
  Delay4/1 -> Bus Creator/3  "in2"
  Delay5/1 -> Bus Creator/4  "in3"
  Delay6/1 -> Bus Creator/5  "in4"
  Delay7/1 -> Bus Creator/6  "in5"
  Delay8/1 -> Bus Creator/7  "in6"
  Delay9/1 -> Bus Creator/8  "in7"
  Delay10/1 -> Bus Creator/9  "in8"
  Delay11/1 -> Bus Creator/10  "in9"
  Delay12/1 -> Bus Creator/11  "in10"
  Delay13/1 -> Bus Creator/12  "in11"
  Delay14/1 -> Bus Creator/13  "in12"
  Delay15/1 -> Bus Creator/14  "in13"
  Delay16/1 -> Bus Creator/15  "in14"
  Delay17/1 -> Bus Creator/16  "in15"
  Delay26/1 -> Bus Creator/17  "in16"
  Delay27/1 -> Bus Creator/18  "in17"
  Delay28/1 -> Bus Creator/19  "in18"
  Delay29/1 -> Bus Creator/20  "in19"
  Delay30/1 -> Bus Creator/21  "in20"
  Delay31/1 -> Bus Creator/22  "in21"
  Delay32/1 -> Bus Creator/23  "in22"
  Delay33/1 -> Bus Creator/24  "in23"
  Delay18/1 -> Bus Creator/25  "in24"
  Delay19/1 -> Bus Creator/26  "in25"
  Delay20/1 -> Bus Creator/27  "in26"
  Delay21/1 -> Bus Creator/28  "in27"
  Delay22/1 -> Bus Creator/29  "in28"
  Delay23/1 -> Bus Creator/30  "in29"
  Delay24/1 -> Bus Creator/31  "in30"
  Delay25/1 -> Bus Creator/32  "in31"
  sel0/1 -> [insel0]
  Constant/1 -> sel0/1
  sel1/1 -> [insel1]
  Constant1/1 -> sel1/1
  sel2/1 -> [insel2]
  Constant2/1 -> sel2/1
  sel3/1 -> [insel3]
  Constant3/1 -> sel3/1
  Delay1/1 -> [pfb_sync]
  mux_0_31/1(out0) -> Delay2/1  "in0"
  mux_0_31/2(out1) -> Delay3/1  "in1"
  mux_0_31/3(out2) -> Delay4/1  "in2"
  mux_0_31/4(out3) -> Delay5/1  "in3"
  mux_0_31/5(out4) -> Delay6/1  "in4"
  mux_0_31/6(out5) -> Delay7/1  "in5"
  mux_0_31/7(out6) -> Delay8/1  "in6"
  mux_0_31/8(out7) -> Delay9/1  "in7"
  mux_0_31/9(out8) -> Delay10/1  "in8"
  mux_0_31/10(out9) -> Delay11/1  "in9"
  mux_0_31/11(out10) -> Delay12/1  "in10"
  mux_0_31/12(out11) -> Delay13/1  "in11"
  mux_0_31/13(out12) -> Delay14/1  "in12"
  mux_0_31/14(out13) -> Delay15/1  "in13"
  mux_0_31/15(out14) -> Delay16/1  "in14"
  mux_0_31/16(out15) -> Delay17/1  "in15"
  mux_0_31/17(out16) -> Delay26/1  "in16"
  mux_0_31/18(out17) -> Delay27/1  "in17"
  mux_0_31/19(out18) -> Delay28/1  "in18"
  mux_0_31/20(out19) -> Delay29/1  "in19"
  mux_0_31/21(out20) -> Delay30/1  "in20"
  mux_0_31/22(out21) -> Delay31/1  "in21"
  mux_0_31/23(out22) -> Delay32/1  "in22"
  mux_0_31/24(out23) -> Delay33/1  "in23"
  mux_0_31/25(out24) -> Delay18/1  "in24"
  mux_0_31/26(out25) -> Delay19/1  "in25"
  mux_0_31/27(out26) -> Delay20/1  "in26"
  mux_0_31/28(out27) -> Delay21/1  "in27"
  mux_0_31/29(out28) -> Delay22/1  "in28"
  mux_0_31/30(out29) -> Delay23/1  "in29"
  mux_0_31/31(out30) -> Delay24/1  "in30"
  mux_0_31/32(out31) -> Delay25/1  "in31"

== system roach2_fengine_nlb/monitor ==
  note: GPIO Select (sync_out)
      | 0: zero
      | 1: sync_gpio_in
      | 2: sync_in
      | 3: adc_clip
      | 4: eq_clip
  note: LED Select
      | 0: Clip (LED1=adc_clip; LED0=eq_clip
      | 1: Sync (LED1=sync_gpio_in; LED0=sync_in)
  note: sel[4] = ledsel
      | sel[2:0] = gpiosel
  BitBasher : xbsIndex_r4/BitBasher  bitexpr=|  display_expr=off  sr_1=1  arith_type1=Unsigned  bin_pt1=0  sr_2=2  arith_type2=Unsigned  bin_pt2=0  sr_3=3  arith_type3=Unsigned  bin_pt3=0  sr_4=4  arith_type4=Unsigned  bin_pt4=0  dbl_ovrd=off  block_type=bitbasher
      | <!DOCTYPE HTML PUBLIC "-//W3C//DTD HTML 4.0//EN" "http://www.w3.org/TR/REC-html40/strict.dtd">
      | <html><head><meta name="qrichtext" content="1" /><style type="text/css">
      | p, li { white-space: pre-wrap; }
      | </style></head><body style=" font-family:'Sans'; font-size:10pt; font-weight:400; font-style:normal;">
      | <p style=" margin-top:12px; margin-bottom:12px; margin-left:0px; margin-right:0px; -qt-block-indent:0; text-indent:0px;"><span style=" font-family:'MS Shell Dlg'; font-size:8pt;">gpiosel={sel[2:0]}<br />ledsel={sel[4]}</span></p></body></html>
  Constant1 : Constant  Value=0
  gpio : Subsystem
  led : Subsystem
  sel : xps_library/software register  Tag=xps:sw_reg  io_dir=From Processor  arith_type=Unsigned  bitwidth=32  bin_pt=0  sample_period=1  gw_name=roach2_fengine_monitor_sel_user_data_out
  wires:
  Constant1/1 -> sel/1
  sel/1 -> BitBasher/1
  BitBasher/1 -> [gpiosel]
  BitBasher/2 -> [ledsel]
  [gpiosel] -> gpio/1(sel)
  [ledsel] -> led/1(sel)

== system roach2_fengine_nlb/noise ==
  Bus Creator : BusCreator  Inputs=32
  noise0 : Subsystem
  noise1 : Subsystem
  noise10 : Subsystem
  noise11 : Subsystem
  noise12 : Subsystem
  noise13 : Subsystem
  noise14 : Subsystem
  noise15 : Subsystem
  noise2 : Subsystem
  noise3 : Subsystem
  noise4 : Subsystem
  noise5 : Subsystem
  noise6 : Subsystem
  noise7 : Subsystem
  noise8 : Subsystem
  noise9 : Subsystem
  Out1 : Outport
  wires:
  noise0/1(n1) -> Bus Creator/1  "n0"
  noise0/2(n2) -> Bus Creator/2  "n1"
  noise1/1(n1) -> Bus Creator/3  "n2"
  noise1/2(n2) -> Bus Creator/4  "n3"
  noise2/1(n1) -> Bus Creator/5  "n4"
  noise2/2(n2) -> Bus Creator/6  "n5"
  noise3/1(n1) -> Bus Creator/7  "n6"
  noise3/2(n2) -> Bus Creator/8  "n7"
  [seed0] -> noise0/1(seed)
  [seed3] -> noise3/1(seed)
  [seed2] -> noise2/1(seed)
  [seed1] -> noise1/1(seed)
  [seed_ld] -> noise0/2(ld)
  [seed_ld] -> noise3/2(ld)
  [seed_ld] -> noise2/2(ld)
  [seed_ld] -> noise1/2(ld)
  Bus Creator/1 -> Out1/1
  noise4/1(n1) -> Bus Creator/9  "n8"
  noise4/2(n2) -> Bus Creator/10  "n9"
  noise5/1(n1) -> Bus Creator/11  "n10"
  noise5/2(n2) -> Bus Creator/12  "n11"
  noise6/1(n1) -> Bus Creator/13  "n12"
  noise6/2(n2) -> Bus Creator/14  "n13"
  noise7/1(n1) -> Bus Creator/15  "n14"
  noise7/2(n2) -> Bus Creator/16  "n15"
  [seed4] -> noise4/1(seed)
  [seed7] -> noise7/1(seed)
  [seed6] -> noise6/1(seed)
  [seed5] -> noise5/1(seed)
  [seed_ld] -> noise4/2(ld)
  [seed_ld] -> noise7/2(ld)
  [seed_ld] -> noise6/2(ld)
  [seed_ld] -> noise5/2(ld)
  noise8/1(n1) -> Bus Creator/17  "n16"
  noise8/2(n2) -> Bus Creator/18  "n17"
  noise9/1(n1) -> Bus Creator/19  "n18"
  noise9/2(n2) -> Bus Creator/20  "n19"
  noise10/1(n1) -> Bus Creator/21  "n20"
  noise10/2(n2) -> Bus Creator/22  "n21"
  noise11/1(n1) -> Bus Creator/23  "n22"
  noise11/2(n2) -> Bus Creator/24  "n23"
  [seed8] -> noise8/1(seed)
  [seed11] -> noise11/1(seed)
  [seed10] -> noise10/1(seed)
  [seed9] -> noise9/1(seed)
  [seed_ld] -> noise8/2(ld)
  [seed_ld] -> noise11/2(ld)
  [seed_ld] -> noise10/2(ld)
  [seed_ld] -> noise9/2(ld)
  noise12/1(n1) -> Bus Creator/25  "n24"
  noise12/2(n2) -> Bus Creator/26  "n25"
  noise13/1(n1) -> Bus Creator/27  "n26"
  noise13/2(n2) -> Bus Creator/28  "n27"
  noise14/1(n1) -> Bus Creator/29  "n28"
  noise14/2(n2) -> Bus Creator/30  "n29"
  noise15/1(n1) -> Bus Creator/31  "n30"
  noise15/2(n2) -> Bus Creator/32  "n31"
  [seed12] -> noise12/1(seed)
  [seed15] -> noise15/1(seed)
  [seed14] -> noise14/1(seed)
  [seed13] -> noise13/1(seed)
  [seed_ld] -> noise12/2(ld)
  [seed_ld] -> noise15/2(ld)
  [seed_ld] -> noise14/2(ld)
  [seed_ld] -> noise13/2(ld)

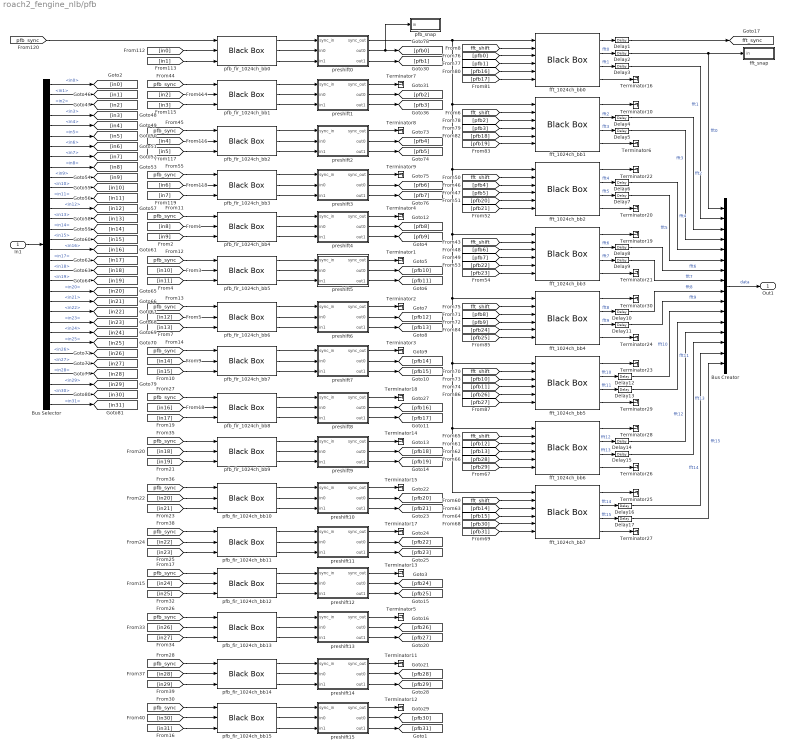
== system roach2_fengine_nlb/pfb ==
  In1 : Inport
  Bus Creator : BusCreator  Inputs=16
  Bus Selector : BusSelector  OutputSignals=in0,in1,in2,in3,in4,in5,in6,in7,in8,in9,in10,in11,in12,in13,in14,in15,in16,in17,in18,in19,in20,in21,in22,in23,in24,in25,in26,in27,in28,in29,in30,in31
  Delay{1..17} (17 alike) : xbsIndex_r4/Delay  rst=off  infoeditControl=Selection of Reset will increase slice count due to use of real FFs and instead of SRLs  en=off  latency=1  dbl_ovrd=off  reg_retiming=off  block_type=delay
  Terminator{1..30} (30 alike) : Terminator
  fft_1024ch_bb{0..7} (8 alike) : xbsIndex_r4/Black Box  init_code=fft_1024ch_core_config  sim_method=Inactive  verbose=off  block_type=blackbox2
  fft_snap : Subsystem
  pfb_fir_1024ch_bb{0..15} (16 alike) : xbsIndex_r4/Black Box  init_code=pfb_fir_1024ch_core_config  sim_method=Inactive  verbose=off  block_type=blackbox2
  pfb_snap : Subsystem
  preshift0 : Subsystem
  preshift1 : Subsystem
  preshift10 : Subsystem
  preshift11 : Subsystem
  preshift12 : Subsystem
  preshift13 : Subsystem
  preshift14 : Subsystem
  preshift15 : Subsystem
  preshift2 : Subsystem
  preshift3 : Subsystem
  preshift4 : Subsystem
  preshift5 : Subsystem
  preshift6 : Subsystem
  preshift7 : Subsystem
  preshift8 : Subsystem
  preshift9 : Subsystem
  Out1 : Outport
  tag scope: fft_sync=global
  wires:
  [in0] -> pfb_fir_1024ch_bb0/2
  [in1] -> pfb_fir_1024ch_bb0/3
  [in2] -> pfb_fir_1024ch_bb1/2
  [in3] -> pfb_fir_1024ch_bb1/3
  [in4] -> pfb_fir_1024ch_bb2/2
  [in5] -> pfb_fir_1024ch_bb2/3
  [in6] -> pfb_fir_1024ch_bb3/2
  [in7] -> pfb_fir_1024ch_bb3/3
  pfb_fir_1024ch_bb1/2 -> preshift1/2(in0)
  pfb_fir_1024ch_bb1/3 -> preshift1/3(in1)
  pfb_fir_1024ch_bb2/2 -> preshift2/2(in0)
  pfb_fir_1024ch_bb2/3 -> preshift2/3(in1)
  pfb_fir_1024ch_bb3/2 -> preshift3/2(in0)
  pfb_fir_1024ch_bb3/3 -> preshift3/3(in1)
  [fft_shift] -> fft_1024ch_bb1/2
  fft_1024ch_bb1/4 -> Terminator6/1
  fft_1024ch_bb0/4 -> Terminator16/1
  Delay1/1 -> [fft_sync]
  fft_1024ch_bb1/1 -> Terminator10/1
  [fft_shift] -> fft_1024ch_bb0/2
  [pfb_sync] -> pfb_fir_1024ch_bb0/1
  [pfb_sync] -> pfb_fir_1024ch_bb1/1
  [pfb_sync] -> pfb_fir_1024ch_bb2/1
  [pfb_sync] -> pfb_fir_1024ch_bb3/1
  pfb_fir_1024ch_bb1/1 -> preshift1/1(sync_in)
  pfb_fir_1024ch_bb2/1 -> preshift2/1(sync_in)
  pfb_fir_1024ch_bb3/1 -> preshift3/1(sync_in)
  pfb_fir_1024ch_bb0/1 -> preshift0/1(sync_in)
  pfb_fir_1024ch_bb0/2 -> preshift0/2(in0)
  pfb_fir_1024ch_bb0/3 -> preshift0/3(in1)
  preshift0/1(sync_out) -> fft_1024ch_bb6/1, fft_1024ch_bb7/1, fft_1024ch_bb5/1, fft_1024ch_bb4/1, fft_1024ch_bb3/1, fft_1024ch_bb2/1, fft_1024ch_bb1/1, fft_1024ch_bb0/1
  preshift0/2(out0) -> [pfb0], pfb_snap/1(in)
  preshift0/3(out1) -> [pfb1]
  preshift1/1(sync_out) -> Terminator7/1
  preshift2/1(sync_out) -> Terminator8/1
  preshift3/1(sync_out) -> Terminator9/1
  preshift1/2(out0) -> [pfb2]
  preshift1/3(out1) -> [pfb3]
  preshift2/2(out0) -> [pfb4]
  preshift2/3(out1) -> [pfb5]
  preshift3/2(out0) -> [pfb6]
  preshift3/3(out1) -> [pfb7]
  [pfb0] -> fft_1024ch_bb0/3
  [pfb1] -> fft_1024ch_bb0/4
  [pfb16] -> fft_1024ch_bb0/5
  [pfb17] -> fft_1024ch_bb0/6
  [pfb2] -> fft_1024ch_bb1/3
  [pfb3] -> fft_1024ch_bb1/4
  [pfb18] -> fft_1024ch_bb1/5
  [pfb19] -> fft_1024ch_bb1/6
  [in8] -> pfb_fir_1024ch_bb4/2
  [in9] -> pfb_fir_1024ch_bb4/3
  [in10] -> pfb_fir_1024ch_bb5/2
  [in11] -> pfb_fir_1024ch_bb5/3
  [in12] -> pfb_fir_1024ch_bb6/2
  [in13] -> pfb_fir_1024ch_bb6/3
  [in14] -> pfb_fir_1024ch_bb7/2
  [in15] -> pfb_fir_1024ch_bb7/3
  pfb_fir_1024ch_bb5/2 -> preshift5/2(in0)
  pfb_fir_1024ch_bb5/3 -> preshift5/3(in1)
  pfb_fir_1024ch_bb6/2 -> preshift6/2(in0)
  pfb_fir_1024ch_bb6/3 -> preshift6/3(in1)
  pfb_fir_1024ch_bb7/2 -> preshift7/2(in0)
  pfb_fir_1024ch_bb7/3 -> preshift7/3(in1)
  [pfb_sync] -> pfb_fir_1024ch_bb4/1
  [pfb_sync] -> pfb_fir_1024ch_bb5/1
  [pfb_sync] -> pfb_fir_1024ch_bb6/1
  [pfb_sync] -> pfb_fir_1024ch_bb7/1
  pfb_fir_1024ch_bb5/1 -> preshift5/1(sync_in)
  pfb_fir_1024ch_bb6/1 -> preshift6/1(sync_in)
  pfb_fir_1024ch_bb7/1 -> preshift7/1(sync_in)
  pfb_fir_1024ch_bb4/1 -> preshift4/1(sync_in)
  pfb_fir_1024ch_bb4/2 -> preshift4/2(in0)
  pfb_fir_1024ch_bb4/3 -> preshift4/3(in1)
  preshift4/1(sync_out) -> Terminator4/1
  preshift4/2(out0) -> [pfb8]
  preshift4/3(out1) -> [pfb9]
  preshift5/1(sync_out) -> Terminator1/1
  preshift6/1(sync_out) -> Terminator2/1
  preshift7/1(sync_out) -> Terminator3/1
  preshift5/2(out0) -> [pfb10]
  preshift5/3(out1) -> [pfb11]
  preshift6/2(out0) -> [pfb12]
  preshift6/3(out1) -> [pfb13]
  preshift7/2(out0) -> [pfb14]
  preshift7/3(out1) -> [pfb15]
  [in16] -> pfb_fir_1024ch_bb8/2
  [in17] -> pfb_fir_1024ch_bb8/3
  [in18] -> pfb_fir_1024ch_bb9/2
  [in19] -> pfb_fir_1024ch_bb9/3
  [in20] -> pfb_fir_1024ch_bb10/2
  [in21] -> pfb_fir_1024ch_bb10/3
  [in22] -> pfb_fir_1024ch_bb11/2
  [in23] -> pfb_fir_1024ch_bb11/3
  pfb_fir_1024ch_bb9/2 -> preshift9/2(in0)
  pfb_fir_1024ch_bb9/3 -> preshift9/3(in1)
  pfb_fir_1024ch_bb10/2 -> preshift10/2(in0)
  pfb_fir_1024ch_bb10/3 -> preshift10/3(in1)
  pfb_fir_1024ch_bb11/2 -> preshift11/2(in0)
  pfb_fir_1024ch_bb11/3 -> preshift11/3(in1)
  [pfb_sync] -> pfb_fir_1024ch_bb8/1
  [pfb_sync] -> pfb_fir_1024ch_bb9/1
  [pfb_sync] -> pfb_fir_1024ch_bb10/1
  [pfb_sync] -> pfb_fir_1024ch_bb11/1
  pfb_fir_1024ch_bb9/1 -> preshift9/1(sync_in)
  pfb_fir_1024ch_bb10/1 -> preshift10/1(sync_in)
  pfb_fir_1024ch_bb11/1 -> preshift11/1(sync_in)
  pfb_fir_1024ch_bb8/1 -> preshift8/1(sync_in)
  pfb_fir_1024ch_bb8/2 -> preshift8/2(in0)
  pfb_fir_1024ch_bb8/3 -> preshift8/3(in1)
  preshift8/1(sync_out) -> Terminator18/1
  preshift8/2(out0) -> [pfb16]
  preshift8/3(out1) -> [pfb17]
  preshift9/1(sync_out) -> Terminator14/1
  preshift10/1(sync_out) -> Terminator15/1
  preshift11/1(sync_out) -> Terminator17/1
  preshift9/2(out0) -> [pfb18]
  preshift9/3(out1) -> [pfb19]
  preshift10/2(out0) -> [pfb20]
  preshift10/3(out1) -> [pfb21]
  preshift11/2(out0) -> [pfb22]
  preshift11/3(out1) -> [pfb23]
  [in24] -> pfb_fir_1024ch_bb12/2
  [in25] -> pfb_fir_1024ch_bb12/3
  [in26] -> pfb_fir_1024ch_bb13/2
  [in27] -> pfb_fir_1024ch_bb13/3
  [in28] -> pfb_fir_1024ch_bb14/2
  [in29] -> pfb_fir_1024ch_bb14/3
  [in30] -> pfb_fir_1024ch_bb15/2
  [in31] -> pfb_fir_1024ch_bb15/3
  pfb_fir_1024ch_bb13/2 -> preshift13/2(in0)
  pfb_fir_1024ch_bb13/3 -> preshift13/3(in1)
  pfb_fir_1024ch_bb14/2 -> preshift14/2(in0)
  pfb_fir_1024ch_bb14/3 -> preshift14/3(in1)
  pfb_fir_1024ch_bb15/2 -> preshift15/2(in0)
  pfb_fir_1024ch_bb15/3 -> preshift15/3(in1)
  [pfb_sync] -> pfb_fir_1024ch_bb12/1
  [pfb_sync] -> pfb_fir_1024ch_bb13/1
  [pfb_sync] -> pfb_fir_1024ch_bb14/1
  [pfb_sync] -> pfb_fir_1024ch_bb15/1
  pfb_fir_1024ch_bb13/1 -> preshift13/1(sync_in)
  pfb_fir_1024ch_bb14/1 -> preshift14/1(sync_in)
  pfb_fir_1024ch_bb15/1 -> preshift15/1(sync_in)
  pfb_fir_1024ch_bb12/1 -> preshift12/1(sync_in)
  pfb_fir_1024ch_bb12/2 -> preshift12/2(in0)
  pfb_fir_1024ch_bb12/3 -> preshift12/3(in1)
  preshift12/1(sync_out) -> Terminator13/1
  preshift12/2(out0) -> [pfb24]
  preshift12/3(out1) -> [pfb25]
  preshift13/1(sync_out) -> Terminator5/1
  preshift14/1(sync_out) -> Terminator11/1
  preshift15/1(sync_out) -> Terminator12/1
  preshift13/2(out0) -> [pfb26]
  preshift13/3(out1) -> [pfb27]
  preshift14/2(out0) -> [pfb28]
  preshift14/3(out1) -> [pfb29]
  preshift15/2(out0) -> [pfb30]
  preshift15/3(out1) -> [pfb31]
  [fft_shift] -> fft_1024ch_bb3/2
  fft_1024ch_bb3/4 -> Terminator21/1
  fft_1024ch_bb2/4 -> Terminator20/1
  fft_1024ch_bb2/1 -> Terminator22/1
  fft_1024ch_bb3/1 -> Terminator19/1
  [fft_shift] -> fft_1024ch_bb2/2
  [pfb4] -> fft_1024ch_bb2/3
  [pfb5] -> fft_1024ch_bb2/4
  [pfb20] -> fft_1024ch_bb2/5
  [pfb21] -> fft_1024ch_bb2/6
  [pfb6] -> fft_1024ch_bb3/3
  [pfb7] -> fft_1024ch_bb3/4
  [pfb22] -> fft_1024ch_bb3/5
  [pfb23] -> fft_1024ch_bb3/6
  [fft_shift] -> fft_1024ch_bb5/2
  fft_1024ch_bb5/4 -> Terminator29/1
  fft_1024ch_bb4/4 -> Terminator24/1
  fft_1024ch_bb4/1 -> Terminator30/1
  fft_1024ch_bb5/1 -> Terminator23/1
  [fft_shift] -> fft_1024ch_bb4/2
  [pfb8] -> fft_1024ch_bb4/3
  [pfb9] -> fft_1024ch_bb4/4
  [pfb24] -> fft_1024ch_bb4/5
  [pfb25] -> fft_1024ch_bb4/6
  [pfb10] -> fft_1024ch_bb5/3
  [pfb11] -> fft_1024ch_bb5/4
  [pfb26] -> fft_1024ch_bb5/5
  [pfb27] -> fft_1024ch_bb5/6
  [fft_shift] -> fft_1024ch_bb7/2
  fft_1024ch_bb7/4 -> Terminator27/1
  fft_1024ch_bb6/4 -> Terminator26/1
  fft_1024ch_bb6/1 -> Terminator28/1
  fft_1024ch_bb7/1 -> Terminator25/1
  [fft_shift] -> fft_1024ch_bb6/2
  [pfb12] -> fft_1024ch_bb6/3
  [pfb13] -> fft_1024ch_bb6/4
  [pfb28] -> fft_1024ch_bb6/5
  [pfb29] -> fft_1024ch_bb6/6
  [pfb14] -> fft_1024ch_bb7/3
  [pfb15] -> fft_1024ch_bb7/4
  [pfb30] -> fft_1024ch_bb7/5
  [pfb31] -> fft_1024ch_bb7/6
  In1/1 -> Bus Selector/1
  Bus Selector/1 -> [in0]  "<in0>"
  Bus Selector/2 -> [in1]  "<in1>"
  Bus Selector/3 -> [in2]  "<in2>"
  Bus Selector/4 -> [in3]  "<in3>"
  Bus Selector/5 -> [in4]  "<in4>"
  Bus Selector/6 -> [in5]  "<in5>"
  Bus Selector/7 -> [in6]  "<in6>"
  Bus Selector/8 -> [in7]  "<in7>"
  Bus Selector/9 -> [in8]  "<in8>"
  Bus Selector/10 -> [in9]  "<in9>"
  Bus Selector/11 -> [in10]  "<in10>"
  Bus Selector/12 -> [in11]  "<in11>"
  Bus Selector/13 -> [in12]  "<in12>"
  Bus Selector/14 -> [in13]  "<in13>"
  Bus Selector/15 -> [in14]  "<in14>"
  Bus Selector/16 -> [in15]  "<in15>"
  Bus Selector/17 -> [in16]  "<in16>"
  Bus Selector/18 -> [in17]  "<in17>"
  Bus Selector/19 -> [in18]  "<in18>"
  Bus Selector/20 -> [in19]  "<in19>"
  Bus Selector/21 -> [in20]  "<in20>"
  Bus Selector/22 -> [in21]  "<in21>"
  Bus Selector/23 -> [in22]  "<in22>"
  Bus Selector/24 -> [in23]  "<in23>"
  Bus Selector/25 -> [in24]  "<in24>"
  Bus Selector/26 -> [in25]  "<in25>"
  Bus Selector/27 -> [in26]  "<in26>"
  Bus Selector/28 -> [in27]  "<in27>"
  Bus Selector/29 -> [in28]  "<in28>"
  Bus Selector/30 -> [in29]  "<in29>"
  Bus Selector/31 -> [in30]  "<in30>"
  Bus Selector/32 -> [in31]  "<in31>"
  Delay2/1 -> Bus Creator/1, fft_snap/1(in)  "fft0"
  Delay3/1 -> Bus Creator/2  "fft1"
  Delay4/1 -> Bus Creator/3  "fft2"
  Delay5/1 -> Bus Creator/4  "fft3"
  Delay6/1 -> Bus Creator/5  "fft4"
  Delay7/1 -> Bus Creator/6  "fft5"
  Delay8/1 -> Bus Creator/7  "fft6"
  Delay9/1 -> Bus Creator/8  "fft7"
  Delay10/1 -> Bus Creator/9  "fft8"
  Delay11/1 -> Bus Creator/10  "fft9"
  Delay12/1 -> Bus Creator/11  "fft10"
  Delay13/1 -> Bus Creator/12  "fft11"
  Delay14/1 -> Bus Creator/13  "fft12"
  Delay15/1 -> Bus Creator/14  "fft13"
  Delay16/1 -> Bus Creator/15  "fft14"
  Delay17/1 -> Bus Creator/16  "fft15"
  Bus Creator/1 -> Out1/1  "data"
  fft_1024ch_bb7/2 -> Delay16/1  "fft14"
  fft_1024ch_bb7/3 -> Delay17/1  "fft15"
  fft_1024ch_bb6/2 -> Delay14/1  "fft12"
  fft_1024ch_bb6/3 -> Delay15/1  "fft13"
  fft_1024ch_bb5/2 -> Delay12/1  "fft10"
  fft_1024ch_bb5/3 -> Delay13/1  "fft11"
  fft_1024ch_bb0/2 -> Delay2/1  "fft0"
  fft_1024ch_bb0/1 -> Delay1/1
  fft_1024ch_bb0/3 -> Delay3/1  "fft1"
  fft_1024ch_bb1/2 -> Delay4/1  "fft2"
  fft_1024ch_bb1/3 -> Delay5/1  "fft3"
  fft_1024ch_bb2/2 -> Delay6/1  "fft4"
  fft_1024ch_bb2/3 -> Delay7/1  "fft5"
  fft_1024ch_bb3/2 -> Delay8/1  "fft6"
  fft_1024ch_bb3/3 -> Delay9/1  "fft7"
  fft_1024ch_bb4/2 -> Delay10/1  "fft8"
  fft_1024ch_bb4/3 -> Delay11/1  "fft9"
